simulink model "drone_obs_prev_version"  (R2020a)
settings: Solver=VariableStepAuto  StartTime=0.0  StopTime=20  RelTol=1e-3
undefined symbols (not defined in the file): a1, a2, a3
settings Model: Creator=dfcpstage6  LastModifiedBy=dfcpstage6
settings DebuggingCC: SFMachineParentedDataDiag=error

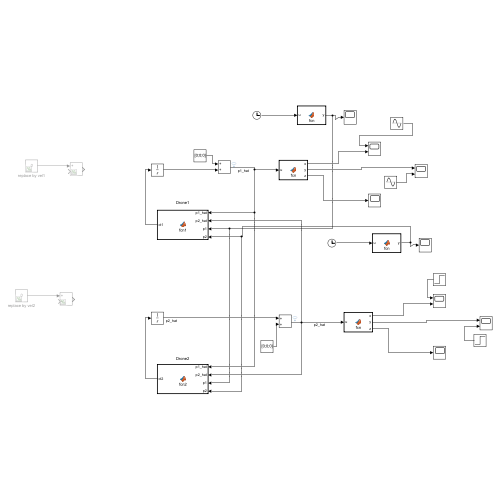
[thumbnail: Simulink's stored preview of the top-level diagram]
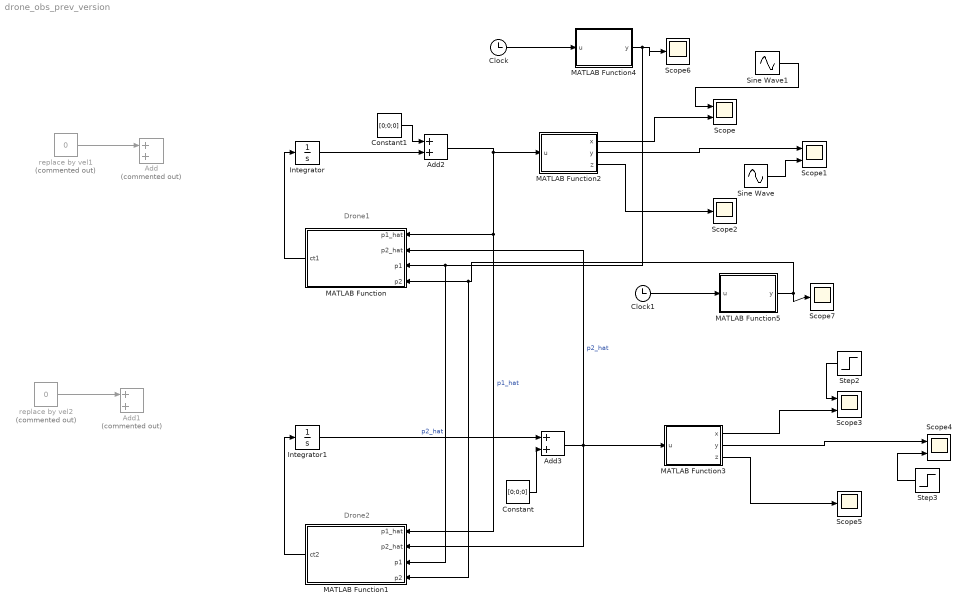
== system drone_obs_prev_version ==
  note: Drone2
  note: Drone1
  Add : Sum  Commented=on
  Add1 : Sum  Commented=on
  Add2 : Sum
  Add3 : Sum
  Clock : Clock
  Clock1 : Clock
  Constant : Constant  Value=[0;0;0]  VectorParams1D=off
  Constant1 : Constant  Value=[0;0;0]  VectorParams1D=off
  Integrator : Integrator
  Integrator1 : Integrator
  MATLAB Function : MATLAB Function  TreatAsAtomicUnit=on
  MATLAB Function1 : MATLAB Function  TreatAsAtomicUnit=on
  MATLAB Function2 : MATLAB Function  TreatAsAtomicUnit=on
  MATLAB Function3 : MATLAB Function  TreatAsAtomicUnit=on
  MATLAB Function4 : MATLAB Function  TreatAsAtomicUnit=on  SystemSampleTime=0.1
  MATLAB Function5 : MATLAB Function  TreatAsAtomicUnit=on  SystemSampleTime=0.1
  Scope{,1,3..4} (4 alike) : Scope  NumInputPorts=2
  Scope{2,5..7} (4 alike) : Scope
  Sine Wave : Sin  SampleTime=0
  Sine Wave1 : Sin  Phase=1.57  SampleTime=0
  Step2 : Step  Time=0.1  After=2  SampleTime=0
  Step3 : Step  Time=0.1  After=2  SampleTime=0
  replace by vel1 : Constant  Commented=on  Value=0
  replace by vel2 : Constant  Commented=on  Value=0
  wires:
  replace by vel1/1 -> Add/1
  replace by vel2/1 -> Add1/1
  MATLAB Function/1(ct1) -> Integrator/1
  MATLAB Function1/1(ct2) -> Integrator1/1
  Integrator/1 -> Add2/2
  Add2/1 -> MATLAB Function1/1(p1_hat), MATLAB Function/1(p1_hat), MATLAB Function2/1(u)  "p1_hat"
  Integrator1/1 -> Add3/1  "p2_hat"
  Constant/1 -> Add3/2
  Constant1/1 -> Add2/1
  MATLAB Function2/2(y) -> Scope1/1
  MATLAB Function2/3(z) -> Scope2/1
  MATLAB Function2/1(x) -> Scope/2
  MATLAB Function5/1(y) -> MATLAB Function1/4(p2), MATLAB Function/4(p2), Scope7/1
  MATLAB Function4/1(y) -> MATLAB Function1/3(p1), MATLAB Function/3(p1), Scope6/1
  MATLAB Function3/2(y) -> Scope4/1
  MATLAB Function3/3(z) -> Scope5/1
  Step2/1 -> Scope3/1
  Step3/1 -> Scope4/2
  MATLAB Function3/1(x) -> Scope3/2
  Add3/1 -> MATLAB Function3/1(u), MATLAB Function1/2(p2_hat), MATLAB Function/2(p2_hat)  "p2_hat"
  Clock/1 -> MATLAB Function4/1(u)
  Clock1/1 -> MATLAB Function5/1(u)
  Sine Wave1/1 -> Scope/1
  Sine Wave/1 -> Scope1/2

== matlab function drone_obs_prev_version/MATLAB Function1 ==
  data: p1_hat input; p2_hat input; ct2 output; a2 parameter; a3 parameter; p1 input; p2 input; a1 parameter
function ct2 = fcn2(p1_hat, p2_hat,a2, a3, p1, p2, a1)

%     a1(1)
    vel2 = [0;0;0];
    d11 = norm(p1-a1);
    d13 = norm(p1-a3);
    d22 = norm(p2-a2);
    d23 = norm(p2-a3);
    q12 = norm(p1-p2);
    q21 = norm(p1-p2);
    y12 = d22^2 - d23^2 + norm(a3)^2 - norm(a2)^2;
    y22 = d23^2 + d13^2 - q21^2 - 2*norm(a3)^2;
    c23 = a3 - a2;
    k12 = c23;
    k22 = p1_hat - a3;
    ct2_1 = k12*(y12 - 2*(c23.')*p2_hat); 
    ct2_2 = k22*(y22 + 2*(a3.')*(p1_hat + p2_hat) - 2*(p1_hat.')*(p2_hat));
ct2 = vel2 + (ct2_1 + ct2_2);

== matlab function drone_obs_prev_version/MATLAB Function ==
  data: p1_hat input; p2_hat input; ct1 output; p1 input; p2 input; a1 parameter; a2 parameter; a3 parameter
% function ct1 = fcn1(p1_hat, p2_hat ,a1, a3, d11, d13, d23, q21)
% 
% %     a1(1)
%     vel1 = [0;0;0];
%     y11 = d11^2 - d13^2 + norm(a3)^2 - norm(a1)^2;
%     y21 = d23^2 + d13^2 - q21^2 - 2*norm(a3)^2;
%     c13 = a3 - a1;
%     k11 = c13; k21 = p2_hat - a3;
%     ct1_1 = k11*(y11 - 2*(c13.')*p1_hat);
%     ct1_2 = k21*(y21 + 2*(a3.')*(p1_hat + p2_hat) - 2*(p1_hat.')*(p2_hat));
%         
%     N = ndims(ct1_1)
% ct1 = vel1 + ct1_1 + ct1_2;

function ct1 = fcn1(p1_hat, p2_hat ,p1, p2, a1, a2, a3)

%     a1(1)
    vel1 = [0;0;0];
    d11 = norm(p1-a1);
    d13 = norm(p1-a3);
    d22 = norm(p2-a2);
    d23 = norm(p2-a3);
    q12 = norm(p1-p2);
    q21 = norm(p1-p2);
    y11 = d11^2 - d13^2 + norm(a3)^2 - norm(a1)^2;
    y21 = d23^2 + d13^2 - q21^2 - 2*norm(a3)^2;
    c13 = a3 - a1;
    k11 = c13; k21 = p2_hat - a3;
    ct1_1 = k11*(y11 - 2*(c13.')*p1_hat);
    ct1_2 = k21*(y21 + 2*(a3.')*(p1_hat + p2_hat) - 2*(p1_hat.')*(p2_hat));
        
    N = ndims(ct1_1)
ct1 = vel1 + ct1_1 + ct1_2;

== matlab function drone_obs_prev_version/MATLAB Function2 ==
  data: u input; x output; y output; z output; xunit parameter
function [x,y,z]= fcn(u, xunit)
%     x = u(1);
    x = u(1);
    y = u(2);
    z = u(3);
% y = u;

== matlab function drone_obs_prev_version/MATLAB Function3 ==
  data: u input; x output; y output; z output
function [x,y,z]= fcn(u)
    x = u(1);
    y = u(2);
    z = u(3);
% y = u;

== matlab function drone_obs_prev_version/MATLAB Function4 ==
  data: y output; u input
function y = fcn(u)
    t = linspace(0,5);
    xc = cos(u);
    yc = sin(u);
y = [xc;yc;0];

== matlab function drone_obs_prev_version/MATLAB Function5 ==
  data: y output; u input
function y = fcn(u)
    t = linspace(0,5);
    xc = sin(u);
% y = xc;
y = [2;2;0];
